simulink model "prob1_week_3"  (R2020b)
settings: Solver=VariableStepAuto  StartTime=0.0  StopTime=10.0  RelTol=1e-3
settings Model: Creator=Pulkit Khandelwal  LastModifiedBy=Pulkit Khandelwal

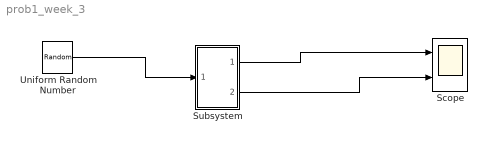
== system prob1_week_3 ==
  Scope : Scope  NumInputPorts=2
  Subsystem : Subsystem  TreatAsAtomicUnit=on
  Uniform Random Number : UniformRandomNumber  Minimum=0  Maximum=2  Seed=337  SampleTime=5
  wires:
  Uniform Random Number/1 -> Subsystem/1(In1)
  Subsystem/1(Coin) -> Scope/1
  Subsystem/2(data) -> Scope/2

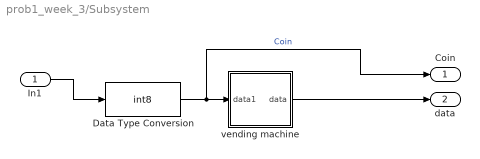
== system prob1_week_3/Subsystem ==
  In1 : Inport
  Data Type Conversion : DataTypeConversion  OutDataTypeStr=int8  RndMeth=Nearest  SaturateOnIntegerOverflow=on
  vending machine : Stateflow chart  TreatAsAtomicUnit=on
  Coin : Outport
  data : Outport  Port=2
  wires:
  Data Type Conversion/1 -> Coin/1, vending machine/1(data1)  "Coin"
  In1/1 -> Data Type Conversion/1
  vending machine/1(data) -> data/1

== stateflow chart prob1_week_3/Subsystem/vending machine ==
  settings: stateMachineType=MEALY_MACHINE
  state Got_0
  state Got_Nickel
  state Got_Dime
  (default) -> Got_0
  Got_0 -> Got_Nickel [order 1] : [data1==1]{data=0}
  Got_Nickel -> Got_0 [order 1] : [data1==2]{data=1}
  Got_Dime -> Got_0 [order 2] : [data1==1]{data=1}
  Got_0 -> Got_Dime [order 2] : [data1==2]{data=0}
  Got_Nickel -> Got_Dime [order 2] : [data1==1]{data=0}
  Got_Dime -> Got_Nickel [order 1] : [data1==2]{data=1}
  data: data output; data1 input
